simulink model "paper_Exponential_Predefined_102"  (R2019a)
settings: Solver=ode4  StartTime=0.0  StopTime=40  FixedStep=0.001  RelTol=1e-3
libraries: simulink x6
(part 1 of 3)
settings Model: Creator=maple  LastModifiedBy=maple

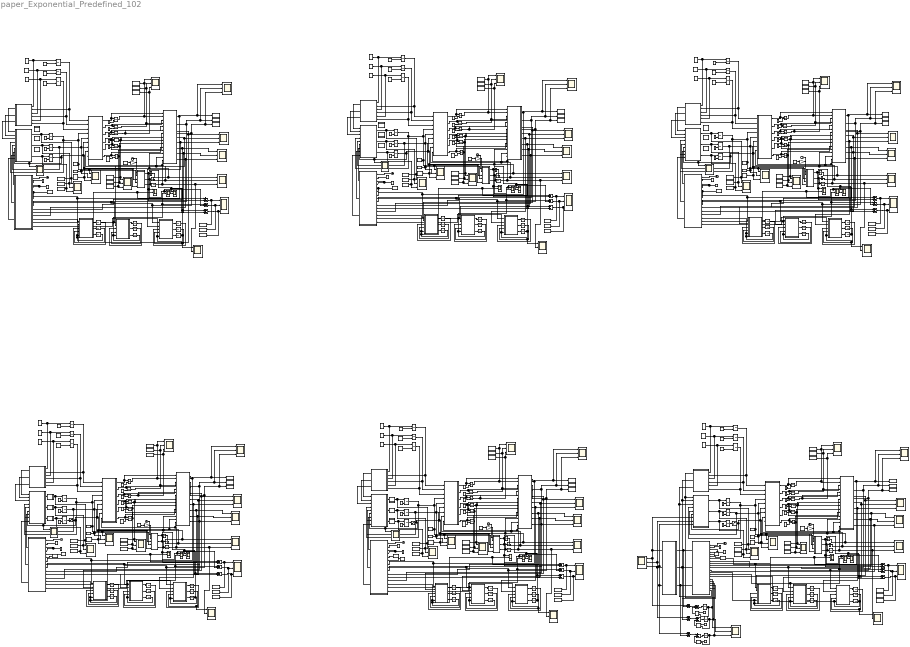
== system paper_Exponential_Predefined_102 ==
  note: p1z
  note: p2y
  note: p2z
  note: Predefined time in paper[11]
  note: p1x
  note: p2x
  note: p1y
  note: p1z
  note: p2z
  note: p1x
  note: Exponential predefined time
      | [This paper]
  note: p2y
  note: p2x
  note: p1y
  note: p1z
  note: p2z
  note: p1x
  note: p2y
  note: p2x
  note: p1y
  note: p2x
  note: tua1
  note: p1x
  note: p2z
  note: tua3
  note: p2y
  note: tua2
  note: p1y
  note: p1z
  note: p1y
  note: p2z
  note: p1z
  note: p1x
  note: Exponential
  note: p2x
  note: p2y
  note: p1z
  note: p2y
  note: p1x
  note: p2z
  note: p2x
  note: p1y
  note: Predefined time in paper[11]
  note: Exponential
  note: Exponential predefined time
      | [This paper]
  note: Without input saturation and disturbance
  note: With input saturation and disturbance
  " a^r1" : MATLAB Function  TreatAsAtomicUnit=on
  " a^r2" : MATLAB Function  TreatAsAtomicUnit=on
  " a^r3" : MATLAB Function  TreatAsAtomicUnit=on
  " a^r4" : MATLAB Function  TreatAsAtomicUnit=on
  " a^r5" : MATLAB Function  TreatAsAtomicUnit=on
  Add{1..15,39..47} (24 alike) : Sum  Inputs=+-
  Band-Limited White Noise{1..6} (6 alike) : simulink/Sources/Band-Limited White Noise  Cov=0.01  Ts=0.01  seed=[23341]
  Clock{1..6} (6 alike) : Clock
  Gain{1..6} (6 alike) : Gain  Gain=0.05
  MATLAB Function1 : MATLAB Function  TreatAsAtomicUnit=on
  MATLAB Function10 : MATLAB Function  TreatAsAtomicUnit=on
  MATLAB Function11 : MATLAB Function  TreatAsAtomicUnit=on
  MATLAB Function12 : MATLAB Function  TreatAsAtomicUnit=on
  MATLAB Function13 : MATLAB Function  TreatAsAtomicUnit=on
  MATLAB Function14 : MATLAB Function  TreatAsAtomicUnit=on
  MATLAB Function15 : MATLAB Function  TreatAsAtomicUnit=on
  MATLAB Function16 : MATLAB Function  TreatAsAtomicUnit=on
  MATLAB Function17 : MATLAB Function  TreatAsAtomicUnit=on
  MATLAB Function18 : MATLAB Function  TreatAsAtomicUnit=on
  MATLAB Function19 : MATLAB Function  TreatAsAtomicUnit=on
  MATLAB Function2 : MATLAB Function  TreatAsAtomicUnit=on
  MATLAB Function20 : MATLAB Function  TreatAsAtomicUnit=on
  MATLAB Function21 : MATLAB Function  TreatAsAtomicUnit=on
  MATLAB Function22 : MATLAB Function  TreatAsAtomicUnit=on
  MATLAB Function23 : MATLAB Function  TreatAsAtomicUnit=on
  MATLAB Function24 : MATLAB Function  TreatAsAtomicUnit=on
  MATLAB Function3 : MATLAB Function  TreatAsAtomicUnit=on
  MATLAB Function4 : MATLAB Function  TreatAsAtomicUnit=on
  MATLAB Function5 : MATLAB Function  TreatAsAtomicUnit=on
  MATLAB Function6 : MATLAB Function  TreatAsAtomicUnit=on
  MATLAB Function7 : MATLAB Function  TreatAsAtomicUnit=on
  MATLAB Function8 : MATLAB Function  TreatAsAtomicUnit=on
  MATLAB Function9 : MATLAB Function  TreatAsAtomicUnit=on
  Product13 : Product
  Product14 : Product
  Product15 : Product
  To Workspace1 : ToWorkspace  VariableName=deta  SampleTime=-1
  To Workspace10 : ToWorkspace  VariableName=x  SampleTime=-1
  To Workspace100 : ToWorkspace  VariableName=deta15  SampleTime=-1
  To Workspace101 : ToWorkspace  VariableName=y5  SampleTime=-1
  To Workspace102 : ToWorkspace  VariableName=p1x5  SampleTime=-1
  To Workspace103 : ToWorkspace  VariableName=p1y5  SampleTime=-1
  To Workspace104 : ToWorkspace  VariableName=xr5  SampleTime=-1
  To Workspace105 : ToWorkspace  VariableName=p1z5  SampleTime=-1
  To Workspace106 : ToWorkspace  VariableName=yr5  SampleTime=-1
  To Workspace107 : ToWorkspace  VariableName=z5  SampleTime=-1
  To Workspace108 : ToWorkspace  VariableName=zr5  SampleTime=-1
  To Workspace11 : ToWorkspace  VariableName=u  SampleTime=-1
  To Workspace12 : ToWorkspace  VariableName=u1  SampleTime=-1
  To Workspace13 : ToWorkspace  VariableName=u2  SampleTime=-1
  To Workspace14 : ToWorkspace  VariableName=psi  SampleTime=-1
  To Workspace15 : ToWorkspace  VariableName=gamma  SampleTime=-1
  To Workspace16 : ToWorkspace  VariableName=v  SampleTime=-1
  To Workspace17 : ToWorkspace  VariableName=deta1  SampleTime=-1
  To Workspace18 : ToWorkspace  VariableName=deta2  SampleTime=-1
  To Workspace19 : ToWorkspace  VariableName=deta3  SampleTime=-1
  To Workspace2 : ToWorkspace  VariableName=y  SampleTime=-1
  To Workspace20 : ToWorkspace  VariableName=x1  SampleTime=-1
  To Workspace21 : ToWorkspace  VariableName=u3  SampleTime=-1
  To Workspace22 : ToWorkspace  VariableName=u4  SampleTime=-1
  To Workspace23 : ToWorkspace  VariableName=u5  SampleTime=-1
  To Workspace24 : ToWorkspace  VariableName=psi1  SampleTime=-1
  To Workspace25 : ToWorkspace  VariableName=gamma1  SampleTime=-1
  To Workspace26 : ToWorkspace  VariableName=v1  SampleTime=-1
  To Workspace27 : ToWorkspace  VariableName=deta4  SampleTime=-1
  To Workspace28 : ToWorkspace  VariableName=deta5  SampleTime=-1
  To Workspace29 : ToWorkspace  VariableName=y1  SampleTime=-1
  To Workspace3 : ToWorkspace  VariableName=p1x  SampleTime=-1
  To Workspace30 : ToWorkspace  VariableName=p1x1  SampleTime=-1
  To Workspace31 : ToWorkspace  VariableName=p1y1  SampleTime=-1
  To Workspace32 : ToWorkspace  VariableName=xr1  SampleTime=-1
  To Workspace33 : ToWorkspace  VariableName=p1z1  SampleTime=-1
  To Workspace34 : ToWorkspace  VariableName=yr1  SampleTime=-1
  To Workspace35 : ToWorkspace  VariableName=z1  SampleTime=-1
  To Workspace36 : ToWorkspace  VariableName=zr1  SampleTime=-1
  To Workspace37 : ToWorkspace  VariableName=deta6  SampleTime=-1
  To Workspace38 : ToWorkspace  VariableName=x2  SampleTime=-1
  To Workspace39 : ToWorkspace  VariableName=u6  SampleTime=-1
  To Workspace4 : ToWorkspace  VariableName=p1y  SampleTime=-1
  To Workspace40 : ToWorkspace  VariableName=u7  SampleTime=-1
  To Workspace41 : ToWorkspace  VariableName=u8  SampleTime=-1
  To Workspace42 : ToWorkspace  VariableName=psi2  SampleTime=-1
  To Workspace43 : ToWorkspace  VariableName=gamma2  SampleTime=-1
  To Workspace44 : ToWorkspace  VariableName=v2  SampleTime=-1
  To Workspace45 : ToWorkspace  VariableName=deta7  SampleTime=-1
  To Workspace46 : ToWorkspace  VariableName=deta8  SampleTime=-1
  To Workspace47 : ToWorkspace  VariableName=y2  SampleTime=-1
  To Workspace48 : ToWorkspace  VariableName=p1x2  SampleTime=-1
  To Workspace49 : ToWorkspace  VariableName=p1y2  SampleTime=-1
  To Workspace5 : ToWorkspace  VariableName=xr  SampleTime=-1
  To Workspace50 : ToWorkspace  VariableName=xr2  SampleTime=-1
  To Workspace51 : ToWorkspace  VariableName=p1z2  SampleTime=-1
  To Workspace52 : ToWorkspace  VariableName=yr2  SampleTime=-1
  To Workspace53 : ToWorkspace  VariableName=z2  SampleTime=-1
  To Workspace54 : ToWorkspace  VariableName=zr2  SampleTime=-1
  To Workspace55 : ToWorkspace  VariableName=deta9  SampleTime=-1
  To Workspace56 : ToWorkspace  VariableName=x3  SampleTime=-1
  To Workspace57 : ToWorkspace  VariableName=u9  SampleTime=-1
  To Workspace58 : ToWorkspace  VariableName=u10  SampleTime=-1
  To Workspace59 : ToWorkspace  VariableName=u11  SampleTime=-1
  To Workspace6 : ToWorkspace  VariableName=p1z  SampleTime=-1
  To Workspace60 : ToWorkspace  VariableName=psi3  SampleTime=-1
  To Workspace61 : ToWorkspace  VariableName=gamma3  SampleTime=-1
  To Workspace62 : ToWorkspace  VariableName=v3  SampleTime=-1
  To Workspace63 : ToWorkspace  VariableName=deta10  SampleTime=-1
  To Workspace64 : ToWorkspace  VariableName=deta11  SampleTime=-1
  To Workspace65 : ToWorkspace  VariableName=y3  SampleTime=-1
  To Workspace66 : ToWorkspace  VariableName=p1x3  SampleTime=-1
  To Workspace67 : ToWorkspace  VariableName=p1y3  SampleTime=-1
  To Workspace68 : ToWorkspace  VariableName=xr3  SampleTime=-1
  To Workspace69 : ToWorkspace  VariableName=p1z3  SampleTime=-1
  To Workspace7 : ToWorkspace  VariableName=yr  SampleTime=-1
  To Workspace70 : ToWorkspace  VariableName=yr3  SampleTime=-1
  To Workspace71 : ToWorkspace  VariableName=z3  SampleTime=-1
  To Workspace72 : ToWorkspace  VariableName=zr3  SampleTime=-1
  To Workspace73 : ToWorkspace  VariableName=deta12  SampleTime=-1
  To Workspace74 : ToWorkspace  VariableName=x4  SampleTime=-1
  To Workspace75 : ToWorkspace  VariableName=u12  SampleTime=-1
  To Workspace76 : ToWorkspace  VariableName=u13  SampleTime=-1
  To Workspace77 : ToWorkspace  VariableName=u14  SampleTime=-1
  To Workspace78 : ToWorkspace  VariableName=psi4  SampleTime=-1
  To Workspace79 : ToWorkspace  VariableName=gamma4  SampleTime=-1
  To Workspace8 : ToWorkspace  VariableName=z  SampleTime=-1
  To Workspace80 : ToWorkspace  VariableName=v4  SampleTime=-1
  To Workspace81 : ToWorkspace  VariableName=deta13  SampleTime=-1
  To Workspace82 : ToWorkspace  VariableName=deta14  SampleTime=-1
  To Workspace83 : ToWorkspace  VariableName=y4  SampleTime=-1
  To Workspace84 : ToWorkspace  VariableName=p1x4  SampleTime=-1
  To Workspace85 : ToWorkspace  VariableName=p1y4  SampleTime=-1
  To Workspace86 : ToWorkspace  VariableName=xr4  SampleTime=-1
  To Workspace87 : ToWorkspace  VariableName=p1z4  SampleTime=-1
  To Workspace88 : ToWorkspace  VariableName=yr4  SampleTime=-1
  To Workspace89 : ToWorkspace  VariableName=z4  SampleTime=-1
  To Workspace9 : ToWorkspace  VariableName=zr  SampleTime=-1
  To Workspace90 : ToWorkspace  VariableName=zr4  SampleTime=-1
  To Workspace91 : ToWorkspace  VariableName=x5  SampleTime=-1
  To Workspace92 : ToWorkspace  VariableName=u15  SampleTime=-1
  To Workspace93 : ToWorkspace  VariableName=u16  SampleTime=-1
  To Workspace94 : ToWorkspace  VariableName=u17  SampleTime=-1
  To Workspace95 : ToWorkspace  VariableName=psi5  SampleTime=-1
  To Workspace96 : ToWorkspace  VariableName=gamma5  SampleTime=-1
  To Workspace97 : ToWorkspace  VariableName=v5  SampleTime=-1
  To Workspace98 : ToWorkspace  VariableName=deta16  SampleTime=-1
  To Workspace99 : ToWorkspace  VariableName=deta17  SampleTime=-1
  U : MATLAB Function  TreatAsAtomicUnit=on
  X{1..5} (5 alike) : Scope  NumInputPorts=3
  X_dot1 : MATLAB Function  TreatAsAtomicUnit=on
  X_dot2 : MATLAB Function  TreatAsAtomicUnit=on
  X_dot3 : MATLAB Function  TreatAsAtomicUnit=on
  X_dot4 : MATLAB Function  TreatAsAtomicUnit=on
  X_dot5 : MATLAB Function  TreatAsAtomicUnit=on
  X_dot6 : MATLAB Function  TreatAsAtomicUnit=on
  ar{1..6} (6 alike) : Constant  Value=0
  bta{1..6} (6 alike) : Constant  Value=6
  control input 1 : MATLAB Function  TreatAsAtomicUnit=on
  control input 2 : MATLAB Function  TreatAsAtomicUnit=on
  control input 3 : MATLAB Function  TreatAsAtomicUnit=on
  control input 4 : MATLAB Function  TreatAsAtomicUnit=on
  control input 5 : MATLAB Function  TreatAsAtomicUnit=on
  d2x {1..6} (6 alike) : Integrator
  d2y {1..6} (6 alike) : Integrator
  d2z {1..6} (6 alike) : Integrator
  error_FTDO1 : Scope  NumInputPorts=3
  error_FTDO2 : Scope  NumInputPorts=3
  f,df1 : MATLAB Function  TreatAsAtomicUnit=on
  f,df2 : MATLAB Function  TreatAsAtomicUnit=on
  f,df3 : MATLAB Function  TreatAsAtomicUnit=on
  f,df4 : MATLAB Function  TreatAsAtomicUnit=on
  f,df5 : MATLAB Function  TreatAsAtomicUnit=on
  gamma{1,3,5,7,9,11} (6 alike) : Constant  Value=0
  gamma{2,4,6,8,10,12} (6 alike) : Integrator  InitialConditionSource=external
  gamma_r{1,3,5,7,9,11} (6 alike) : Integrator  InitialConditionSource=external
  gamma_r{2,4,6,8,10,12} (6 alike) : Constant  Value=0.2
  k{1..2,4..5,8,18} (6 alike) : Constant
  k19 : Constant  Value=3
  k20 : Constant  Value=3
  k21 : Constant  Value=3
  k3 : Constant  Value=0.3
  k7 : Constant  Value=0.3
  k9 : Constant  Value=0.3
  omiga__gamma_r{1..6} (6 alike) : Constant  Value=0
  omiga_psi_r{1..6} (6 alike) : Constant  Value=0.3
  p{1..28,35..36} (30 alike) : Scope  NumInputPorts=3
  predefined : MATLAB Function  TreatAsAtomicUnit=on
  psi{1,3,5,7,9,11} (6 alike) : Constant  Value=0
  psi{2,4,6,8,10,12} (6 alike) : Integrator  InitialConditionSource=external
  psi_r{1,3,5,7,9} (5 alike) : Constant  Value=3.14/4
  psi_r{2,4,6,8,10,12} (6 alike) : Integrator  InitialConditionSource=external
  psi_r11 : Constant  Value=0.3
  qnta : MATLAB Function  TreatAsAtomicUnit=on
  real_disturbance : Scope  NumInputPorts=3
  ref_UAV : MATLAB Function  TreatAsAtomicUnit=on
  reference_position : Scope  NumInputPorts=3
  sat_v1 : Saturate  UpperLimit=30  LowerLimit=10
  sat_v2 : Saturate  UpperLimit=30  LowerLimit=10
  sat_v6 : Saturate  UpperLimit=40  LowerLimit=10
  show Xr{1..5} (5 alike) : Scope  NumInputPorts=3
  show_p1 : Scope  NumInputPorts=3
  show_p2 : Scope  NumInputPorts=3
  show_qnta : Scope  NumInputPorts=3
  show_s : Scope  NumInputPorts=3
  show_tua : Scope  NumInputPorts=3
  show_u{,1..10} (11 alike) : Scope  NumInputPorts=3
  show_v psi gamma{1..24} (24 alike) : Scope  NumInputPorts=3
  sys : MATLAB Function  TreatAsAtomicUnit=on
  t{1..6} (6 alike) : Clock
  t_f1 : Constant  Value=5
  t_f2 : Constant  Value=5
  t_f3 : Constant  Value=20
  t_f4 : Constant  Value=5
  t_f5 : Constant  Value=20
  t_f6 : Constant  Value=20
  tua13 : Integrator
  tua14 : Integrator
  tua15 : Integrator
  u_1a1 : MATLAB Function  TreatAsAtomicUnit=on
  u_1a2 : MATLAB Function  TreatAsAtomicUnit=on
  u_1a3 : MATLAB Function  TreatAsAtomicUnit=on
  u_1a4 : MATLAB Function  TreatAsAtomicUnit=on
  u_1a5 : MATLAB Function  TreatAsAtomicUnit=on
  u_2a1 : MATLAB Function  TreatAsAtomicUnit=on
  u_2a2 : MATLAB Function  TreatAsAtomicUnit=on
  u_2a3 : MATLAB Function  TreatAsAtomicUnit=on
  u_2a4 : MATLAB Function  TreatAsAtomicUnit=on
  u_2a6 : MATLAB Function  TreatAsAtomicUnit=on
  u_3a1 : MATLAB Function  TreatAsAtomicUnit=on
  u_3a2 : MATLAB Function  TreatAsAtomicUnit=on
  u_3a3 : MATLAB Function  TreatAsAtomicUnit=on
  u_3a4 : MATLAB Function  TreatAsAtomicUnit=on
  u_3a5 : MATLAB Function  TreatAsAtomicUnit=on
  uav_position : Scope  NumInputPorts=3
  v{1,3,5,7,9,11} (6 alike) : Constant  Value=10
  v{2,4,6,8,10,12} (6 alike) : Integrator  InitialConditionSource=external
  vr{1,3,5,7,9,11} (6 alike) : Constant  Value=20
  vr{2,4,6,8,10,12} (6 alike) : Integrator  InitialConditionSource=external
  x{1,3,5,7,9,11} (6 alike) : Constant  Value=0
  x{2,4,6,8,10,12} (6 alike) : Integrator  InitialConditionSource=external
  xr{1,3,5,7,9,11} (6 alike) : Constant  Value=70
  xr{2,4,6,8,10,12} (6 alike) : Integrator  InitialConditionSource=external
  y{1,3,5,7,9,11} (6 alike) : Constant  Value=0
  y{2,4,6,8,10,12} (6 alike) : Integrator  InitialConditionSource=external
  yr{1,3,5,7,9,11} (6 alike) : Constant  Value=90
  yr{2,4,6,8,10,12} (6 alike) : Integrator  InitialConditionSource=external
  yuding_zhishu1 : MATLAB Function  TreatAsAtomicUnit=on
  yuding_zhishu2 : MATLAB Function  TreatAsAtomicUnit=on
  yuding_zhishu3 : MATLAB Function  TreatAsAtomicUnit=on
  yuding_zhishu4 : MATLAB Function  TreatAsAtomicUnit=on
  yuding_zhishu5 : MATLAB Function  TreatAsAtomicUnit=on
  z0x{1..6} (6 alike) : Integrator  InitialCondition=70
  z0y{1..6} (6 alike) : Integrator  InitialCondition=90
  z0z{1..6} (6 alike) : Integrator  InitialCondition=-100
  z{1,3,5,7,9,11} (6 alike) : Constant  Value=0
  z{2,4,6,8,10,12} (6 alike) : Integrator  InitialConditionSource=external
  z1x{1..6} (6 alike) : Integrator
  z1y{1..6} (6 alike) : Integrator
  z1z{1..6} (6 alike) : Integrator
  z2x{1..6} (6 alike) : Integrator
  z2y{1..6} (6 alike) : Integrator
  z2z{1..6} (6 alike) : Integrator
  zr{1,3,5,7,9,11} (6 alike) : Constant  Value=-100
  zr{2,4,6,8,10,12} (6 alike) : Integrator  InitialConditionSource=external
  wires:
  yr2/1 -> To Workspace7/1, show Xr1/2, f,df1/10(yr)
  zr2/1 -> To Workspace9/1, show Xr1/3, f,df1/12(zr)
  MATLAB Function1/1(dz0y) -> z0y1/1
  d2y 1/1 -> p6/2, f,df1/14(wy), X_dot1/8(wy)
  MATLAB Function4/1(dz0x) -> z0x1/1
  t1/1 -> yuding_zhishu1/1(t)
  " a^r1"/1(a_xr) -> control input 1/1(a_xr)
  omiga__gamma_r1/1 -> " a^r1"/5(omiga_gamma_r), gamma_r1/1
  f,df1/2(p1y) -> MATLAB Function1/1(p1y), yuding_zhishu1/8(p1y), To Workspace4/1, p4/2
  z0y1/1 -> MATLAB Function1/3(z0y)
  f,df1/5(p2y) -> MATLAB Function1/2(p2y), p5/2
  X_dot1/4(xr_dot) -> f,df1/7(dxr), xr2/1
  Band-Limited White Noise1/1 -> Gain1/1
  x2/1 -> To Workspace10/1, X1/1, f,df1/2(x)
  MATLAB Function3/2(dz1z) -> z1z1/1
  " a^r1"/3(a_zr) -> control input 1/3(a_zr)
  z0x1/1 -> MATLAB Function4/3(z0x)
  d2x 1/1 -> f,df1/13(wx), X_dot1/7(wx), p6/1
  xr1/1 -> xr2/2
  gamma2/1 -> MATLAB Function2/4(gamma), show_v psi gamma4/2, To Workspace15/1, X_dot1/5(gamma), control input 1/5(gamma)
  z2/1 -> To Workspace8/1, X1/3, f,df1/6(z)
  psi2/1 -> To Workspace14/1, show_v psi gamma4/1, MATLAB Function2/5(psi), X_dot1/4(psi), control input 1/4(psi)
  MATLAB Function4/2(dz1x) -> z1x1/1
  MATLAB Function4/3(dz2x) -> z2x1/1
  MATLAB Function2/1(dx) -> Add3/2, show_v psi gamma1/1, d2x 1/1
  xr2/1 -> To Workspace5/1, show Xr1/1, f,df1/8(xr)
  z1x1/1 -> MATLAB Function4/4(z1x)
  z1y1/1 -> MATLAB Function1/4(z1y)
  bta1/1 -> yuding_zhishu1/4(bta2), yuding_zhishu1/3(bta1)
  k1/1 -> yuding_zhishu1/6(k2), yuding_zhishu1/5(k1)
  z1z1/1 -> MATLAB Function3/4(z1z), p2/1
  X_dot1/1(s1) -> f,df1/1(dx), x2/1
  f,df1/1(p1x) -> MATLAB Function4/1(p1x), yuding_zhishu1/7(p1x), To Workspace3/1, p4/1
  Clock1/1 -> MATLAB Function2/1(t)
  x1/1 -> x2/2
  psi_r1/1 -> psi_r2/2
  gamma_r1/1 -> " a^r1"/6(gamma_r), X_dot1/3(gamma_r)
  z2y1/1 -> MATLAB Function1/5(z2y), Add4/1, show_v psi gamma2/2, yuding_zhishu1/14(z2y)
  f,df1/8(s2) -> yuding_zhishu1/11(p2y), p3/2
  d2z 1/1 -> f,df1/15(wz), X_dot1/9(wz), p2/2, p6/3
  f,df1/3(p1z) -> MATLAB Function3/1(p1z), yuding_zhishu1/9(p1z), To Workspace6/1, p4/3
  Add5/1 -> To Workspace1/1, p1/3
  t_f1/1 -> yuding_zhishu1/2(t_f)
  f,df1/6(p2z) -> MATLAB Function3/2(p2z), p5/3
  X_dot1/6(zr_dot) -> f,df1/11(dzr), zr2/1
  gamma_r2/1 -> gamma_r1/2
  MATLAB Function1/2(dz1y) -> z1y1/1
  z2z1/1 -> Add5/1, show_v psi gamma3/2, MATLAB Function3/5(z2z), yuding_zhishu1/15(z2z)
  X_dot1/5(yr_dot) -> yr2/1, f,df1/9(dyr)
  z2x1/1 -> Add3/1, show_v psi gamma1/2, MATLAB Function4/5(z2x), yuding_zhishu1/13(z2x)
  vr2/1 -> X_dot1/1(vr), " a^r1"/2(vr)
  ar1/1 -> " a^r1"/1(ar), vr2/1
  MATLAB Function2/2(dy) -> d2y 1/1, Add4/2, show_v psi gamma2/1
  psi_r2/1 -> X_dot1/2(psi_r), " a^r1"/4(psi_r)
  omiga_psi_r1/1 -> " a^r1"/3(omiga_psi_r), psi_r2/1
  y2/1 -> To Workspace2/1, X1/2, f,df1/4(y)
  f,df1/4(p2x) -> MATLAB Function4/2(p2x), p5/1
  MATLAB Function3/1(dz0z) -> z0z1/1
  vr1/1 -> vr2/2
  y1/1 -> y2/2
  " a^r1"/2(a_yr) -> control input 1/2(a_yr)
  f,df1/9(s3) -> yuding_zhishu1/12(p2z), p3/3
  psi1/1 -> psi2/2
  z0z1/1 -> MATLAB Function3/3(z0z)
  Add3/1 -> To Workspace17/1, p1/1
  MATLAB Function3/3(dz2z) -> z2z1/1
  v2/1 -> MATLAB Function2/3(v), To Workspace16/1, show_v psi gamma4/3, X_dot1/6(v), show_u2/1, control input 1/6(v)
  z1/1 -> z2/2
  MATLAB Function1/3(dz2y) -> z2y1/1
  yr1/1 -> yr2/2
  v1/1 -> v2/2
  Gain1/1 -> MATLAB Function2/2(delta)
  X_dot1/2(s2) -> y2/1, f,df1/3(dy)
  gamma1/1 -> gamma2/2
  zr1/1 -> zr2/2
  Add4/1 -> To Workspace18/1, p1/2
  X_dot1/3(s3) -> f,df1/5(dz), z2/1
  f,df1/7(s1) -> yuding_zhishu1/10(p2x), p3/1
  MATLAB Function2/3(dz) -> Add5/2, show_v psi gamma3/1, d2z 1/1
  yuding_zhishu1/1(nta_1) -> control input 1/7(nta_1)
  yuding_zhishu1/2(nta_2) -> control input 1/8(nta_2)
  yuding_zhishu1/3(nta_3) -> control input 1/9(nta_3)
  control input 1/3(u3_a) -> v2/1, To Workspace13/1, show_u1/3
  control input 1/2(u2_omiga_gamma) -> To Workspace12/1, show_u1/2, gamma2/1
  control input 1/1(u1_omiga_psi) -> psi2/1, To Workspace11/1, show_u1/1
  gamma_r3/1 -> " a^r2"/6(gamma_r), X_dot2/3(gamma_r)
  z2y2/1 -> Add2/1, show_v psi gamma6/2, yuding_zhishu2/14(z2y), MATLAB Function5/5(z2y)
  psi_r3/1 -> psi_r4/2
  z0x2/1 -> MATLAB Function8/3(z0x)
  MATLAB Function7/3(dz2z) -> z2z2/1
  y4/1 -> To Workspace29/1, X2/2, f,df2/4(y)
  gamma3/1 -> gamma4/2
  control input 2/1(u1_omiga_psi) -> psi4/1, To Workspace21/1, show_u3/1
  v4/1 -> MATLAB Function6/3(v), To Workspace26/1, show_v psi gamma8/3, X_dot2/6(v), show_u4/1, control input 2/6(v)
  f,df2/6(p2z) -> MATLAB Function7/2(p2z), p11/3
  yuding_zhishu2/3(nta_3) -> control input 2/9(nta_3)
  control input 2/2(u2_omiga_gamma) -> To Workspace22/1, show_u3/2, gamma4/1
  f,df2/7(s1) -> yuding_zhishu2/10(p2x), p9/1
  gamma_r4/1 -> gamma_r3/2
  control input 2/3(u3_a) -> v4/1, To Workspace23/1, show_u3/3
  yuding_zhishu2/2(nta_2) -> control input 2/8(nta_2)
  f,df2/8(s2) -> yuding_zhishu2/11(p2y), p9/2
  z3/1 -> z4/2
  Add2/1 -> To Workspace28/1, p7/2
  yuding_zhishu2/1(nta_1) -> control input 2/7(nta_1)
  MATLAB Function6/3(dz) -> Add6/2, show_v psi gamma7/1, d2z 2/1
  yr3/1 -> yr4/2
  zr3/1 -> zr4/2
  z1y2/1 -> MATLAB Function5/4(z1y)
  X_dot2/2(s2) -> y4/1, f,df2/3(dy)
  X_dot2/3(s3) -> f,df2/5(dz), z4/1
  " a^r2"/2(a_yr) -> control input 2/2(a_yr)
  Band-Limited White Noise2/1 -> Gain2/1
  Add6/1 -> To Workspace19/1, p7/3
  y3/1 -> y4/2
  Add1/1 -> To Workspace27/1, p7/1
  Gain2/1 -> MATLAB Function6/2(delta)
  MATLAB Function8/2(dz1x) -> z1x2/1
  f,df2/2(p1y) -> MATLAB Function5/1(p1y), yuding_zhishu2/8(p1y), To Workspace31/1, p10/2
  MATLAB Function5/3(dz2y) -> z2y2/1
  psi3/1 -> psi4/2
  z0z2/1 -> MATLAB Function7/3(z0z)
  z2z2/1 -> Add6/1, show_v psi gamma7/2, yuding_zhishu2/15(z2z), MATLAB Function7/5(z2z)
  f,df2/9(s3) -> yuding_zhishu2/12(p2z), p9/3
  vr3/1 -> vr4/2
  psi_r4/1 -> X_dot2/2(psi_r), " a^r2"/4(psi_r)
  z1z2/1 -> p8/1, MATLAB Function7/4(z1z)
  MATLAB Function6/1(dx) -> Add1/2, show_v psi gamma5/1, d2x 2/1
  MATLAB Function8/3(dz2x) -> z2x2/1
  xr3/1 -> xr4/2
  z0y2/1 -> MATLAB Function5/3(z0y)
  t2/1 -> yuding_zhishu2/1(t)
  MATLAB Function7/2(dz1z) -> z1z2/1
  d2x 2/1 -> f,df2/13(wx), X_dot2/7(wx), p12/1
  MATLAB Function8/1(dz0x) -> z0x2/1
  omiga__gamma_r2/1 -> " a^r2"/5(omiga_gamma_r), gamma_r3/1
  " a^r2"/1(a_xr) -> control input 2/1(a_xr)
  MATLAB Function5/1(dz0y) -> z0y2/1
  yr4/1 -> To Workspace34/1, show Xr2/2, f,df2/10(yr)
  zr4/1 -> To Workspace36/1, show Xr2/3, f,df2/12(zr)
  v3/1 -> v4/2
  bta2/1 -> yuding_zhishu2/4(bta2), yuding_zhishu2/3(bta1)
  d2y 2/1 -> p12/2, f,df2/14(wy), X_dot2/8(wy)
  psi4/1 -> To Workspace24/1, show_v psi gamma8/1, MATLAB Function6/5(psi), X_dot2/4(psi), control input 2/4(psi)
  z1x2/1 -> MATLAB Function8/4(z1x)
  MATLAB Function7/1(dz0z) -> z0z2/1
  z4/1 -> To Workspace35/1, X2/3, f,df2/6(z)
  gamma4/1 -> MATLAB Function6/4(gamma), show_v psi gamma8/2, To Workspace25/1, X_dot2/5(gamma), control input 2/5(gamma)
  " a^r2"/3(a_zr) -> control input 2/3(a_zr)
  X_dot2/6(zr_dot) -> f,df2/11(dzr), zr4/1
  omiga_psi_r2/1 -> " a^r2"/3(omiga_psi_r), psi_r4/1
  f,df2/1(p1x) -> MATLAB Function8/1(p1x), yuding_zhishu2/7(p1x), To Workspace30/1, p10/1
  f,df2/4(p2x) -> MATLAB Function8/2(p2x), p11/1
  X_dot2/1(s1) -> f,df2/1(dx), x4/1
  x3/1 -> x4/2
  z2x2/1 -> Add1/1, show_v psi gamma5/2, yuding_zhishu2/13(z2x), MATLAB Function8/5(z2x)
  X_dot2/4(xr_dot) -> f,df2/7(dxr), xr4/1
  vr4/1 -> X_dot2/1(vr), " a^r2"/2(vr)
  x4/1 -> To Workspace20/1, X2/1, f,df2/2(x)
  xr4/1 -> To Workspace32/1, show Xr2/1, f,df2/8(xr)
  f,df2/3(p1z) -> MATLAB Function7/1(p1z), yuding_zhishu2/9(p1z), To Workspace33/1, p10/3
  X_dot2/5(yr_dot) -> yr4/1, f,df2/9(dyr)
  k2/1 -> yuding_zhishu2/6(k2), yuding_zhishu2/5(k1)
  f,df2/5(p2y) -> MATLAB Function5/2(p2y), p11/2
  Clock2/1 -> MATLAB Function6/1(t)
  t_f2/1 -> yuding_zhishu2/2(t_f)
  ar2/1 -> " a^r2"/1(ar), vr4/1
  MATLAB Function6/2(dy) -> d2y 2/1, Add2/2, show_v psi gamma6/1
  d2z 2/1 -> f,df2/15(wz), X_dot2/9(wz), p8/2, p12/3
  MATLAB Function5/2(dz1y) -> z1y2/1
  gamma_r5/1 -> " a^r3"/6(gamma_r), X_dot3/3(gamma_r)
  z2y3/1 -> Add8/1, show_v psi gamma10/2, yuding_zhishu3/14(z2y), MATLAB Function9/5(z2y)
  psi_r5/1 -> psi_r6/2
  z0x3/1 -> MATLAB Function12/3(z0x)
  MATLAB Function11/3(dz2z) -> z2z3/1
  y6/1 -> To Workspace47/1, X3/2, f,df3/4(y)
  gamma5/1 -> gamma6/2
  control input 3/1(u1_omiga_psi) -> u_1a3/1(u)
  v6/1 -> sat_v1/1
  f,df3/6(p2z) -> MATLAB Function11/2(p2z), p17/3
  yuding_zhishu3/3(nta_3) -> control input 3/9(nta_3)
  control input 3/2(u2_omiga_gamma) -> u_2a3/1(u)
  f,df3/7(s1) -> yuding_zhishu3/10(p2x), p15/1
  gamma_r6/1 -> gamma_r5/2
  control input 3/3(u3_a) -> u_3a3/1(u)
  yuding_zhishu3/2(nta_2) -> control input 3/8(nta_2)
  f,df3/8(s2) -> yuding_zhishu3/11(p2y), p15/2
  z5/1 -> z6/2
  Add8/1 -> To Workspace46/1, p13/2
  yuding_zhishu3/1(nta_1) -> control input 3/7(nta_1)
  MATLAB Function10/3(dz) -> Add9/2, show_v psi gamma11/1, d2z 3/1
  yr5/1 -> yr6/2
  zr5/1 -> zr6/2
  z1y3/1 -> MATLAB Function9/4(z1y)
  X_dot3/2(s2) -> y6/1, f,df3/3(dy)
  X_dot3/3(s3) -> f,df3/5(dz), z6/1
  " a^r3"/2(a_yr) -> control input 3/2(a_yr)
  Band-Limited White Noise3/1 -> Gain3/1
  Add9/1 -> To Workspace37/1, p13/3
  y5/1 -> y6/2
  Add7/1 -> To Workspace45/1, p13/1
  Gain3/1 -> MATLAB Function10/2(delta)
  MATLAB Function12/2(dz1x) -> z1x3/1
  f,df3/2(p1y) -> MATLAB Function9/1(p1y), yuding_zhishu3/8(p1y), To Workspace49/1, p16/2
  MATLAB Function9/3(dz2y) -> z2y3/1
  psi5/1 -> psi6/2
  z0z3/1 -> MATLAB Function11/3(z0z)
  z2z3/1 -> Add9/1, show_v psi gamma11/2, yuding_zhishu3/15(z2z), MATLAB Function11/5(z2z)
  f,df3/9(s3) -> yuding_zhishu3/12(p2z), p15/3
  vr5/1 -> vr6/2
  psi_r6/1 -> X_dot3/2(psi_r), " a^r3"/4(psi_r)
  z1z3/1 -> p14/1, MATLAB Function11/4(z1z)
  MATLAB Function10/1(dx) -> Add7/2, show_v psi gamma9/1, d2x 3/1
  MATLAB Function12/3(dz2x) -> z2x3/1
  xr5/1 -> xr6/2
  z0y3/1 -> MATLAB Function9/3(z0y)
  t3/1 -> yuding_zhishu3/1(t)
  MATLAB Function11/2(dz1z) -> z1z3/1
  d2x 3/1 -> f,df3/13(wx), X_dot3/7(wx), p18/1
  MATLAB Function12/1(dz0x) -> z0x3/1
  omiga__gamma_r3/1 -> " a^r3"/5(omiga_gamma_r), gamma_r5/1
  " a^r3"/1(a_xr) -> control input 3/1(a_xr)
  MATLAB Function9/1(dz0y) -> z0y3/1
  yr6/1 -> To Workspace52/1, show Xr3/2, f,df3/10(yr)
  zr6/1 -> To Workspace54/1, show Xr3/3, f,df3/12(zr)
  v5/1 -> v6/2
  bta3/1 -> yuding_zhishu3/4(bta2), yuding_zhishu3/3(bta1)
  d2y 3/1 -> p18/2, f,df3/14(wy), X_dot3/8(wy)
  psi6/1 -> To Workspace42/1, show_v psi gamma12/1, MATLAB Function10/5(psi), X_dot3/4(psi), control input 3/4(psi)
  z1x3/1 -> MATLAB Function12/4(z1x)
  MATLAB Function11/1(dz0z) -> z0z3/1
  z6/1 -> To Workspace53/1, X3/3, f,df3/6(z)
  gamma6/1 -> MATLAB Function10/4(gamma), show_v psi gamma12/2, To Workspace43/1, X_dot3/5(gamma), control input 3/5(gamma)
  " a^r3"/3(a_zr) -> control input 3/3(a_zr)
  X_dot3/6(zr_dot) -> f,df3/11(dzr), zr6/1
  omiga_psi_r3/1 -> " a^r3"/3(omiga_psi_r), psi_r6/1
  f,df3/1(p1x) -> MATLAB Function12/1(p1x), yuding_zhishu3/7(p1x), To Workspace48/1, p16/1
  f,df3/4(p2x) -> MATLAB Function12/2(p2x), p17/1
  X_dot3/1(s1) -> f,df3/1(dx), x6/1
  x5/1 -> x6/2
  z2x3/1 -> Add7/1, show_v psi gamma9/2, yuding_zhishu3/13(z2x), MATLAB Function12/5(z2x)
  X_dot3/4(xr_dot) -> f,df3/7(dxr), xr6/1
  vr6/1 -> X_dot3/1(vr), " a^r3"/2(vr)
  x6/1 -> To Workspace38/1, X3/1, f,df3/2(x)
  xr6/1 -> To Workspace50/1, show Xr3/1, f,df3/8(xr)
  f,df3/3(p1z) -> MATLAB Function11/1(p1z), yuding_zhishu3/9(p1z), To Workspace51/1, p16/3
  X_dot3/5(yr_dot) -> yr6/1, f,df3/9(dyr)
  k3/1 -> yuding_zhishu3/5(k1)
  f,df3/5(p2y) -> MATLAB Function9/2(p2y), p17/2
  Clock3/1 -> MATLAB Function10/1(t)
  t_f3/1 -> yuding_zhishu3/2(t_f)
  ar3/1 -> " a^r3"/1(ar), vr6/1
  MATLAB Function10/2(dy) -> d2y 3/1, Add8/2, show_v psi gamma10/1
  d2z 3/1 -> f,df3/15(wz), X_dot3/9(wz), p14/2, p18/3
  MATLAB Function9/2(dz1y) -> z1y3/1
  sat_v1/1 -> MATLAB Function10/3(v), To Workspace44/1, show_v psi gamma12/3, X_dot3/6(v), show_u6/1, control input 3/6(v)
  u_3a3/1(u_3a) -> v6/1, To Workspace41/1, show_u5/3
  u_2a3/1(u_2a) -> To Workspace40/1, show_u5/2, gamma6/1
  u_1a3/1(u_1a) -> psi6/1, To Workspace39/1, show_u5/1
  Band-Limited White Noise6/1 -> Gain6/1
  tua15/1 -> Product15/2, show_tua/3, predefined/18(tua3)
  k19/1 -> Product14/1
  Add44/1 -> Add45/1
  psi11/1 -> psi12/2
  Clock6/1 -> MATLAB Function22/1(t)
  vr12/1 -> X_dot6/1(vr), ref_UAV/2(vr)
  z12/1 -> To Workspace107/1, uav_position/3, sys/6(z)
  t6/1 -> predefined/1(t)
  X_dot6/4(xr_dot) -> sys/7(dxr), xr12/1
  Add47/1 -> tua14/1
  X_dot6/6(zr_dot) -> sys/11(dzr), zr12/1
  MATLAB Function21/1(dz0y) -> z0y6/1
  Product15/1 -> Add40/2
  z0z6/1 -> MATLAB Function23/3(z0z)
  zr12/1 -> To Workspace108/1, reference_position/3, sys/12(zr)
  x11/1 -> x12/2
  z0y6/1 -> MATLAB Function21/3(z0y)
  Add43/1 -> To Workspace100/1, error_FTDO1/3
  sys/7(s1) -> show_s/1, predefined/10(p2x)
  t_f6/1 -> predefined/2(t_f)
  y12/1 -> To Workspace101/1, uav_position/2, sys/4(y)
  Add41/1 -> To Workspace98/1, error_FTDO1/1
  sys/4(p2x) -> MATLAB Function24/2(p2x), show_p2/1
  MATLAB Function22/3(dz) -> Add43/2, show_v psi gamma23/1, d2z 5/1
  Add42/1 -> To Workspace99/1, error_FTDO1/2
  Add39/1 -> Add40/1
  Product14/1 -> Add47/2
  MATLAB Function21/3(dz2y) -> z2y6/1
  z1z6/1 -> error_FTDO2/1, MATLAB Function23/4(z1z)
  v12/1 -> sat_v6/1
  d2x 6/1 -> sys/13(wx), X_dot6/7(wx), real_disturbance/1
  ref_UAV/1(a_xr) -> U/1(a_xr), predefined/19(a_xr)
  sys/3(p1z) -> MATLAB Function23/1(p1z), predefined/9(p1z), To Workspace105/1, show_p1/3
  omiga__gamma_r6/1 -> ref_UAV/5(omiga_gamma_r), gamma_r11/1
  v11/1 -> v12/2
  MATLAB Function21/2(dz1y) -> z1y6/1
  y11/1 -> y12/2
  qnta/3(qnta3) -> Add39/1, U/9(qnta_3), show_qnta/3
  k20/1 -> Product13/1
  z1x6/1 -> MATLAB Function24/4(z1x)
  d2z 5/1 -> sys/15(wz), X_dot6/9(wz), error_FTDO2/2, real_disturbance/3
  z11/1 -> z12/2
  Add40/1 -> tua15/1
  MATLAB Function23/3(dz2z) -> z2z6/1
  sys/6(p2z) -> MATLAB Function23/2(p2z), show_p2/3
  Gain6/1 -> MATLAB Function22/2(delta)
  xr11/1 -> xr12/2
  MATLAB Function23/2(dz1z) -> z1z6/1
  gamma11/1 -> gamma12/2
  yr12/1 -> To Workspace106/1, reference_position/2, sys/10(yr)
  X_dot6/2(dy) -> y12/1, sys/3(dy)
  ref_UAV/3(a_zr) -> U/3(a_zr), predefined/21(a_zr)
  vr11/1 -> vr12/2
  predefined/1(nta_1) -> qnta/1(nta1), Add44/2
  d2y 6/1 -> real_disturbance/2, sys/14(wy), X_dot6/8(wy)
  yr11/1 -> yr12/2
  MATLAB Function24/3(dz2x) -> z2x6/1
  qnta/1(qnta1) -> show_qnta/1, Add44/1, U/7(qnta_1)
  psi_r12/1 -> X_dot6/2(psi_r), ref_UAV/4(psi_r)
  U/1(u1_omiga_psi) -> psi12/1, To Workspace92/1, show_u/1
  MATLAB Function24/1(dz0x) -> z0x6/1
  xr12/1 -> To Workspace104/1, reference_position/1, sys/8(xr)
  sat_v6/1 -> MATLAB Function22/3(v), To Workspace97/1, show_v psi gamma24/3, X_dot6/6(v), U/6(v)
  MATLAB Function24/2(dz1x) -> z1x6/1
  bta6/1 -> predefined/4(bta2), predefined/3(bta1)
  sys/5(p2y) -> MATLAB Function21/2(p2y), show_p2/2
  Product13/1 -> Add45/2
  z2x6/1 -> Add41/1, show_v psi gamma21/2, predefined/13(z2x), MATLAB Function24/5(z2x)
  MATLAB Function23/1(dz0z) -> z0z6/1
  ar6/1 -> ref_UAV/1(ar), vr12/1
  tua13/1 -> show_tua/1, predefined/16(tua1), Product13/2
  X_dot6/5(yr_dot) -> yr12/1, sys/9(dyr)
  sys/1(p1x) -> MATLAB Function24/1(p1x), predefined/7(p1x), To Workspace102/1, show_p1/1
  k18/1 -> predefined/6(k2)
  k21/1 -> Product15/1
  Add46/1 -> Add47/1
  Add45/1 -> tua13/1
  psi12/1 -> To Workspace95/1, show_v psi gamma24/1, MATLAB Function22/5(psi), X_dot6/4(psi), U/4(psi)
  tua14/1 -> show_tua/2, predefined/17(tua2), Product14/2
  z0x6/1 -> MATLAB Function24/3(z0x)
  psi_r11/1 -> psi_r12/2
  z2y6/1 -> predefined/14(z2y), Add42/1, show_v psi gamma22/2, MATLAB Function21/5(z2y)
  predefined/3(nta_3) -> Add39/2, qnta/3(nta3)
  sys/8(s2) -> show_s/2, predefined/11(p2y)
  sys/9(s3) -> show_s/3, predefined/12(p2z)
  qnta/2(qnta2) -> Add46/1, show_qnta/2, U/8(qnta_2)
  zr11/1 -> zr12/2
  MATLAB Function22/1(dx) -> Add41/2, show_v psi gamma21/1, d2x 6/1
  gamma_r11/1 -> ref_UAV/6(gamma_r), X_dot6/3(gamma_r)
  z2z6/1 -> Add43/1, show_v psi gamma23/2, predefined/15(z2z), MATLAB Function23/5(z2z)
  X_dot6/3(dz) -> sys/5(dz), z12/1
  omiga_psi_r6/1 -> ref_UAV/3(omiga_psi_r), psi_r12/1
  gamma_r12/1 -> gamma_r11/2
  predefined/2(nta_2) -> Add46/2, qnta/2(nta2)
  U/2(u2_omiga_gamma) -> To Workspace93/1, show_u/2, gamma12/1
  z1y6/1 -> MATLAB Function21/4(z1y)
  U/3(u3_a) -> v12/1, To Workspace94/1, show_u/3
  ref_UAV/2(a_yr) -> U/2(a_yr), predefined/20(a_yr)
  x12/1 -> To Workspace91/1, uav_position/1, sys/2(x)
  gamma12/1 -> MATLAB Function22/4(gamma), show_v psi gamma24/2, To Workspace96/1, X_dot6/5(gamma), U/5(gamma)
  X_dot6/1(dx) -> sys/1(dx), x12/1
  MATLAB Function22/2(dy) -> d2y 6/1, Add42/2, show_v psi gamma22/1
  sys/2(p1y) -> MATLAB Function21/1(p1y), predefined/8(p1y), To Workspace103/1, show_p1/2
  " a^r4"/3(a_zr) -> control input 4/3(a_zr)
  f,df4/7(s1) -> yuding_zhishu4/10(p2x), p21/1
  Add12/1 -> To Workspace55/1, p19/3
  z7/1 -> z8/2
  t4/1 -> yuding_zhishu4/1(t)
  f,df4/5(p2y) -> MATLAB Function13/2(p2y), p23/2
  MATLAB Function16/2(dz1x) -> z1x4/1
  X_dot4/5(yr_dot) -> yr8/1, f,df4/9(dyr)
  z0y4/1 -> MATLAB Function13/3(z0y)
  psi7/1 -> psi8/2
  bta4/1 -> yuding_zhishu4/4(bta2), yuding_zhishu4/3(bta1)
  control input 4/2(u2_omiga_gamma) -> To Workspace58/1, show_u7/2, gamma8/1
  yuding_zhishu4/3(nta_3) -> control input 4/9(nta_3)
  MATLAB Function14/3(dz) -> Add12/2, show_v psi gamma15/1, d2z 4/1
  f,df4/1(p1x) -> MATLAB Function16/1(p1x), yuding_zhishu4/7(p1x), To Workspace66/1, p22/1
  control input 4/3(u3_a) -> v8/1, To Workspace59/1, show_u7/3
  f,df4/9(s3) -> yuding_zhishu4/12(p2z), p21/3
  d2y 4/1 -> p24/2, f,df4/14(wy), X_dot4/8(wy)
  Add11/1 -> To Workspace64/1, p19/2
  Add10/1 -> To Workspace63/1, p19/1
  " a^r4"/2(a_yr) -> control input 4/2(a_yr)
  zr7/1 -> zr8/2
  yr7/1 -> yr8/2
  MATLAB Function15/3(dz2z) -> z2z4/1
  MATLAB Function15/1(dz0z) -> z0z4/1
  ar4/1 -> " a^r4"/1(ar), vr8/1
  f,df4/2(p1y) -> MATLAB Function13/1(p1y), yuding_zhishu4/8(p1y), To Workspace67/1, p22/2
  psi_r8/1 -> X_dot4/2(psi_r), " a^r4"/4(psi_r)
  z8/1 -> To Workspace71/1, X4/3, f,df4/6(z)
  MATLAB Function14/2(dy) -> d2y 4/1, Add11/2, show_v psi gamma14/1
  y7/1 -> y8/2
  vr7/1 -> vr8/2
  z2z4/1 -> Add12/1, show_v psi gamma15/2, MATLAB Function15/5(z2z), yuding_zhishu4/15(z2z)
  vr8/1 -> X_dot4/1(vr), " a^r4"/2(vr)
  z2x4/1 -> Add10/1, show_v psi gamma13/2, MATLAB Function16/5(z2x), yuding_zhishu4/13(z2x)
  f,df4/6(p2z) -> MATLAB Function15/2(p2z), p23/3
  gamma_r8/1 -> gamma_r7/2
  X_dot4/6(zr_dot) -> f,df4/11(dzr), zr8/1
  MATLAB Function14/1(dx) -> Add10/2, show_v psi gamma13/1, d2x 4/1
  z2y4/1 -> MATLAB Function13/5(z2y), Add11/1, show_v psi gamma14/2, yuding_zhishu4/14(z2y)
  gamma_r7/1 -> " a^r4"/6(gamma_r), X_dot4/3(gamma_r)
  Clock4/1 -> MATLAB Function14/1(t)
  X_dot4/1(s1) -> f,df4/1(dx), x8/1
  k4/1 -> yuding_zhishu4/6(k2), yuding_zhishu4/5(k1)
  z1y4/1 -> MATLAB Function13/4(z1y)
  xr8/1 -> To Workspace68/1, show Xr4/1, f,df4/8(xr)
  z1x4/1 -> MATLAB Function16/4(z1x)
  MATLAB Function16/3(dz2x) -> z2x4/1
  gamma8/1 -> MATLAB Function14/4(gamma), show_v psi gamma16/2, To Workspace61/1, X_dot4/5(gamma), control input 4/5(gamma)
  xr7/1 -> xr8/2
  d2x 4/1 -> f,df4/13(wx), X_dot4/7(wx), p24/1
  z0x4/1 -> MATLAB Function16/3(z0x)
  zr8/1 -> To Workspace72/1, show Xr4/3, f,df4/12(zr)
  X_dot4/3(s3) -> f,df4/5(dz), z8/1
  d2z 4/1 -> f,df4/15(wz), X_dot4/9(wz), p20/2, p24/3
  Gain4/1 -> MATLAB Function14/2(delta)
  X_dot4/2(s2) -> y8/1, f,df4/3(dy)
  MATLAB Function13/1(dz0y) -> z0y4/1
  psi8/1 -> To Workspace60/1, show_v psi gamma16/1, MATLAB Function14/5(psi), X_dot4/4(psi), control input 4/4(psi)
  f,df4/8(s2) -> yuding_zhishu4/11(p2y), p21/2
  x7/1 -> x8/2
  control input 4/1(u1_omiga_psi) -> psi8/1, To Workspace57/1, show_u7/1
  z1z4/1 -> MATLAB Function15/4(z1z), p20/1
  yuding_zhishu4/2(nta_2) -> control input 4/8(nta_2)
  psi_r7/1 -> psi_r8/2
  omiga_psi_r4/1 -> " a^r4"/3(omiga_psi_r), psi_r8/1
  z0z4/1 -> MATLAB Function15/3(z0z)
  gamma7/1 -> gamma8/2
  MATLAB Function16/1(dz0x) -> z0x4/1
  f,df4/3(p1z) -> MATLAB Function15/1(p1z), yuding_zhishu4/9(p1z), To Workspace69/1, p22/3
  y8/1 -> To Workspace65/1, X4/2, f,df4/4(y)
  x8/1 -> To Workspace56/1, X4/1, f,df4/2(x)
  f,df4/4(p2x) -> MATLAB Function16/2(p2x), p23/1
  yuding_zhishu4/1(nta_1) -> control input 4/7(nta_1)
  MATLAB Function15/2(dz1z) -> z1z4/1
  v8/1 -> MATLAB Function14/3(v), To Workspace62/1, show_v psi gamma16/3, X_dot4/6(v), show_u8/1, control input 4/6(v)
  MATLAB Function13/3(dz2y) -> z2y4/1
  MATLAB Function13/2(dz1y) -> z1y4/1
  " a^r4"/1(a_xr) -> control input 4/1(a_xr)
  t_f4/1 -> yuding_zhishu4/2(t_f)
  yr8/1 -> To Workspace70/1, show Xr4/2, f,df4/10(yr)
  omiga__gamma_r4/1 -> " a^r4"/5(omiga_gamma_r), gamma_r7/1
  v7/1 -> v8/2
  X_dot4/4(xr_dot) -> f,df4/7(dxr), xr8/1
  Band-Limited White Noise4/1 -> Gain4/1
  MATLAB Function20/2(dz1y) -> z1y5/1
  u_2a6/1(u_2a) -> To Workspace76/1, show_u9/2, gamma10/1
  t_f5/1 -> yuding_zhishu5/2(t_f)
  X_dot5/5(yr_dot) -> yr10/1, f,df5/9(dyr)
  Clock5/1 -> MATLAB Function17/1(t)
  ar5/1 -> " a^r5"/1(ar), vr10/1
  f,df5/5(p2y) -> MATLAB Function20/2(p2y), p35/2
  z2x5/1 -> Add13/1, show_v psi gamma20/2, yuding_zhishu5/13(z2x), MATLAB Function19/5(z2x)
  f,df5/1(p1x) -> MATLAB Function19/1(p1x), yuding_zhishu5/7(p1x), To Workspace84/1, p28/1
  gamma10/1 -> MATLAB Function17/4(gamma), show_v psi gamma19/2, To Workspace79/1, X_dot5/5(gamma), control input 5/5(gamma)
  f,df5/6(p2z) -> MATLAB Function18/2(p2z), p35/3
  psi10/1 -> To Workspace78/1, show_v psi gamma19/1, MATLAB Function17/5(psi), X_dot5/4(psi), control input 5/4(psi)
  omiga__gamma_r5/1 -> " a^r5"/5(omiga_gamma_r), gamma_r9/1
  d2y 5/1 -> p36/2, f,df5/14(wy), X_dot5/8(wy)
  bta5/1 -> yuding_zhishu5/4(bta2), yuding_zhishu5/3(bta1)
  psi_r10/1 -> X_dot5/2(psi_r), " a^r5"/4(psi_r)
  xr10/1 -> To Workspace86/1, show Xr5/1, f,df5/8(xr)
  d2z 6/1 -> f,df5/15(wz), X_dot5/9(wz), p26/2, p36/3
  Add13/1 -> To Workspace81/1, p25/1
  " a^r5"/1(a_xr) -> control input 5/1(a_xr)
  xr9/1 -> xr10/2
  MATLAB Function19/3(dz2x) -> z2x5/1
  MATLAB Function17/1(dx) -> Add13/2, show_v psi gamma20/1, d2x 5/1
  f,df5/8(s2) -> yuding_zhishu5/11(p2y), p27/2
  psi9/1 -> psi10/2
  MATLAB Function19/2(dz1x) -> z1x5/1
  z0z5/1 -> MATLAB Function18/3(z0z)
  " a^r5"/2(a_yr) -> control input 5/2(a_yr)
  Band-Limited White Noise5/1 -> Gain5/1
  gamma_r9/1 -> " a^r5"/6(gamma_r), X_dot5/3(gamma_r)
  MATLAB Function17/3(dz) -> Add15/2, show_v psi gamma18/1, d2z 6/1
  yuding_zhishu5/2(nta_2) -> control input 5/8(nta_2)
  gamma_r10/1 -> gamma_r9/2
  v10/1 -> sat_v2/1
  control input 5/1(u1_omiga_psi) -> u_1a5/1(u)
  y10/1 -> To Workspace83/1, X5/2, f,df5/4(y)
  psi_r9/1 -> psi_r10/2
  z2y5/1 -> Add14/1, show_v psi gamma17/2, yuding_zhishu5/14(z2y), MATLAB Function20/5(z2y)
  Gain5/1 -> MATLAB Function17/2(delta)
  control input 5/3(u3_a) -> u_3a5/1(u)
  X_dot5/3(s3) -> f,df5/5(dz), z10/1
  MATLAB Function18/3(dz2z) -> z2z5/1
  MATLAB Function18/2(dz1z) -> z1z5/1
  MATLAB Function18/1(dz0z) -> z0z5/1
  u_1a5/1(u_1a) -> psi10/1, To Workspace75/1, show_u9/1
  z1z5/1 -> p26/1, MATLAB Function18/4(z1z)
  z0y5/1 -> MATLAB Function20/3(z0y)
  " a^r5"/3(a_zr) -> control input 5/3(a_zr)
  z2z5/1 -> Add15/1, show_v psi gamma18/2, yuding_zhishu5/15(z2z), MATLAB Function18/5(z2z)
  MATLAB Function20/1(dz0y) -> z0y5/1
  x10/1 -> To Workspace74/1, X5/1, f,df5/2(x)
  z0x5/1 -> MATLAB Function19/3(z0x)
  Add15/1 -> To Workspace73/1, p25/3
  X_dot5/2(s2) -> y10/1, f,df5/3(dy)
  X_dot5/4(xr_dot) -> f,df5/7(dxr), xr10/1
  zr10/1 -> To Workspace90/1, show Xr5/3, f,df5/12(zr)
  x9/1 -> x10/2
  X_dot5/6(zr_dot) -> f,df5/11(dzr), zr10/1
  MATLAB Function17/2(dy) -> d2y 5/1, Add14/2, show_v psi gamma17/1
  yuding_zhishu5/3(nta_3) -> control input 5/9(nta_3)
  gamma9/1 -> gamma10/2
  f,df5/4(p2x) -> MATLAB Function19/2(p2x), p35/1
  t5/1 -> yuding_zhishu5/1(t)
  X_dot5/1(s1) -> f,df5/1(dx), x10/1
  Add14/1 -> To Workspace82/1, p25/2
  sat_v2/1 -> MATLAB Function17/3(v), To Workspace80/1, show_v psi gamma19/3, X_dot5/6(v), show_u10/1, control input 5/6(v)
  f,df5/9(s3) -> yuding_zhishu5/12(p2z), p27/3
  omiga_psi_r5/1 -> " a^r5"/3(omiga_psi_r), psi_r10/1
  yr10/1 -> To Workspace88/1, show Xr5/2, f,df5/10(yr)
  MATLAB Function20/3(dz2y) -> z2y5/1
  z1x5/1 -> MATLAB Function19/4(z1x)
  f,df5/7(s1) -> yuding_zhishu5/10(p2x), p27/1
  f,df5/3(p1z) -> MATLAB Function18/1(p1z), yuding_zhishu5/9(p1z), To Workspace87/1, p28/3
  control input 5/2(u2_omiga_gamma) -> u_2a6/1(u)
  u_3a5/1(u_3a) -> v10/1, To Workspace77/1, show_u9/3
  f,df5/2(p1y) -> MATLAB Function20/1(p1y), yuding_zhishu5/8(p1y), To Workspace85/1, p28/2
  vr9/1 -> vr10/2
  yr9/1 -> yr10/2
  y9/1 -> y10/2
  v9/1 -> v10/2
  k5/1 -> yuding_zhishu5/5(k1)
  z10/1 -> To Workspace89/1, X5/3, f,df5/6(z)
  MATLAB Function19/1(dz0x) -> z0x5/1
  z9/1 -> z10/2
  vr10/1 -> X_dot5/1(vr), " a^r5"/2(vr)
  yuding_zhishu5/1(nta_1) -> control input 5/7(nta_1)
  zr9/1 -> zr10/2
  d2x 5/1 -> f,df5/13(wx), X_dot5/7(wx), p36/1
  z1y5/1 -> MATLAB Function20/4(z1y)
  k7/1 -> predefined/5(k1)
  k8/1 -> yuding_zhishu3/6(k2)
  k9/1 -> yuding_zhishu5/6(k2)

== matlab function paper_Exponential_Predefined_102/ a^r1 ==
  data: ar input; vr input; a_xr output; a_yr output; omiga_psi_r input; psi_r input; omiga_gamma_r input; a_zr output; gamma_r input
function [a_xr,a_yr,a_zr] = fcn(ar,vr,omiga_psi_r,psi_r,omiga_gamma_r,gamma_r)
a_xr = -vr*sin(psi_r)*cos(gamma_r)*omiga_psi_r-vr*cos(psi_r)*sin(gamma_r)*omiga_gamma_r+cos(psi_r)*cos(gamma_r)*ar;
a_yr = vr*cos(psi_r)*cos(gamma_r)*omiga_psi_r-vr*sin(psi_r)*sin(gamma_r)*omiga_gamma_r+ sin(psi_r)*cos(gamma_r)*ar;
a_zr = vr*cos(gamma_r)*omiga_gamma_r + sin(gamma_r)*ar;
end

== matlab function paper_Exponential_Predefined_102/MATLAB Function1 ==
  data: p1y input; p2y input; z0y input; dz0y output; dz1y output; dz2y output; z1y input; z2y input
function [dz0y,dz1y,dz2y] = FTDO(p1y,p2y,z0y,z1y,z2y)
r=[24 216 864];
r0=r(1);
r1=r(2);
r2=r(3);
v0=-r0*(abs(z0y-p1y))^(0.8)*sign(z0y-p1y)-r0*(abs(z0y-p1y))^(1.2)*sign(z0y-p1y)+z1y;
dz0y=v0+p2y;
v1=-r1*(abs(z0y-p1y))^(0.6)*sign(z0y-p1y)-r1*(abs(z0y-p1y))^(1.4)*sign(z0y-p1y)+z2y;
dz1y=v1;
dz2y =-r2*(abs(z0y-p1y))^(0.4)*sign(z0y-p1y)-r2*(abs(z0y-p1y))^(1.6)*sign(z0y-p1y);
end

== matlab function paper_Exponential_Predefined_102/MATLAB Function2 ==
  data: t input; dx output; dy output; dz output; delta input; v input; gamma input; psi input
function [dx,dy,dz] = disturbance(t,delta,v,gamma,psi)
fx=-0.0005*abs(v-36)*exp((0.4*v)^0.5)+0.2*sin(psi);
fy=-0.0004*abs(v-30)*exp((0.3*v)^0.5)+0.2*cos(psi);
fz=-0.004*v^(0.5)*sin(3*gamma);
% fx=0;
% fy=0;
% fz=0;
if 0<t && t<10
    wx = 1*sin(t)+delta;
else
    wx=0;
end
if 5<t && t<15
    wy = 2*sin(2*t)-cos(3*t)+delta;
else
    wy=0;
end
if 0<t && t<20
    wz = 0.5*sin(t)+delta;
else
    wz = 0;
end

dx=fx+wx;
dy=fy+wy;
dz=fz+wz;

end

== matlab function paper_Exponential_Predefined_102/MATLAB Function3 ==
  data: p1z input; p2z input; z0z input; dz0z output; dz1z output; dz2z output; z1z input; z2z input
function [dz0z,dz1z,dz2z] = FTDO(p1z,p2z,z0z,z1z,z2z)
r=[24 216 864];
r0=r(1);
r1=r(2);
r2=r(3);
v0=-r0*(abs(z0z-p1z))^(0.8)*sign(z0z-p1z)-r0*(abs(z0z-p1z))^(1.2)*sign(z0z-p1z)+z1z;
dz0z=v0+p2z;
v1=-r1*(abs(z0z-p1z))^(0.6)*sign(z0z-p1z)-r1*(abs(z0z-p1z))^(1.4)*sign(z0z-p1z)+z2z;
dz1z=v1;
dz2z =-r2*(abs(z0z-p1z))^(0.4)*sign(z0z-p1z)-r2*(abs(z0z-p1z))^(1.6)*sign(z0z-p1z);
end

== matlab function paper_Exponential_Predefined_102/MATLAB Function4 ==
  data: p1x input; p2x input; z0x input; dz0x output; dz1x output; dz2x output; z1x input; z2x input
function [dz0x,dz1x,dz2x] = FTDO(p1x,p2x,z0x,z1x,z2x)
r=[24 216 864];%parameters of FTDO
r0=r(1);
r1=r(2);
r2=r(3);
v0=-r0*(abs(z0x-p1x))^(0.8)*sign(z0x-p1x)-r0*(abs(z0x-p1x))^(1.2)*sign(z0x-p1x)+z1x;
dz0x=v0+p2x;
v1=-r1*(abs(z0x-p1x))^(0.6)*sign(z0x-p1x)-r1*(abs(z0x-p1x))^(1.4)*sign(z0x-p1x)+z2x;
dz1x=v1;
dz2x =-r2*(abs(z0x-p1x))^(0.4)*sign(z0x-p1x)-r2*(abs(z0x-p1x))^(1.6)*sign(z0x-p1x);
end

== matlab function paper_Exponential_Predefined_102/X_dot1 ==
  data: vr input; psi_r input; gamma_r input; psi input; gamma input; v input; s1 output; s2 output; s3 output; xr_dot output; yr_dot output; zr_dot output; wx input; wy input; wz input
function [s1,s2,s3,xr_dot,yr_dot,zr_dot] = fcn(vr,psi_r,gamma_r,psi,gamma,v,wx,wy,wz)
wx=0;
wy=0;
wz=0;
s1 = v*cos(psi)*cos(gamma)+wx;
s2 = v*sin(psi)*cos(gamma)+wy;
s3 = v*sin(gamma)+wz;
xr_dot = vr*cos(psi_r)*cos(gamma_r);
yr_dot = vr*sin(psi_r)*cos(gamma_r);
zr_dot = vr*sin(gamma_r);
end

== matlab function paper_Exponential_Predefined_102/control input 1 ==
  data: a_xr input; a_yr input; a_zr input; psi input; gamma input; u1_omiga_psi output; u2_omiga_gamma output; u3_a output; v input; nta_1 input; nta_2 input; nta_3 input
function [u1_omiga_psi,u2_omiga_gamma,u3_a] = fcn(a_xr,a_yr,a_zr,psi,gamma,v,nta_1,nta_2,nta_3)
A = [-a_xr;-a_yr;-a_zr];
B = [-v*sin(psi)*cos(gamma) -v*cos(psi)*sin(gamma) cos(psi)*cos(gamma); 
    v*cos(psi)*cos(gamma) -v*sin(psi)*sin(gamma) sin(psi)*cos(gamma);
    0                        v*cos(gamma)               sin(gamma)];
nta = [nta_1 ; nta_2;nta_3];
U = -inv(B)*(A - nta);
U11=U(1,1); 
U21=U(2,1);
U31=U(3,1);
% 

u1_omiga_psi = U11 ;
u2_omiga_gamma = U21;
u3_a =U31 ;






end

== matlab function paper_Exponential_Predefined_102/f,df1 ==
  data: dx input; x input; dy input; y input; dz input; z input; dxr input; xr input; dyr input; yr input; dzr input; zr input; p1x output; p1y output; p1z output; p2x output; p2y output; p2z output; wx input; wy input; wz input; s1 output; s2 output; s3 output
 function [p1x,p1y,p1z,p2x,p2y,p2z,s1,s2,s3] = fcn(dx,x,dy,y,dz,z,dxr,xr,dyr,yr,dzr,zr,wx,wy,wz)
wx=0;
wy=0;
wz=0;
p1x = x - xr;
p1y = y - yr;
p1z = z - zr;
s1 = dx - dxr ;
s2 = dy - dyr ;
s3 = dz - dzr ;%w为了确保输入的p2是没有包含扰动的，这样估计值才会准
p2x = dx - dxr-wx ;
p2y = dy - dyr-wy ;
p2z = dz - dzr-wz ;
end

== matlab function paper_Exponential_Predefined_102/ a^r2 ==
  data: ar input; vr input; a_xr output; a_yr output; omiga_psi_r input; psi_r input; omiga_gamma_r input; a_zr output; gamma_r input
function [a_xr,a_yr,a_zr] = fcn(ar,vr,omiga_psi_r,psi_r,omiga_gamma_r,gamma_r)
a_xr = -vr*sin(psi_r)*cos(gamma_r)*omiga_psi_r-vr*cos(psi_r)*sin(gamma_r)*omiga_gamma_r+cos(psi_r)*cos(gamma_r)*ar;
a_yr = vr*cos(psi_r)*cos(gamma_r)*omiga_psi_r-vr*sin(psi_r)*sin(gamma_r)*omiga_gamma_r+ sin(psi_r)*cos(gamma_r)*ar;
a_zr = vr*cos(gamma_r)*omiga_gamma_r + sin(gamma_r)*ar;
end

== matlab function paper_Exponential_Predefined_102/u_1a2 ==
  data: u input; u_1a output
function u_1a  = fcn(u)

u_max=1;

u_1a=u_max*erf((pi^(0.5)*u)/(2*u_max));


 end

== matlab function paper_Exponential_Predefined_102/u_2a1 ==
  data: u input; u_2a output
function u_2a  = fcn(u)

u_max=1;

u_2a=u_max*erf((pi^(0.5)*u)/(2*u_max));


 end

== matlab function paper_Exponential_Predefined_102/u_3a1 ==
  data: u input; u_3a output
function u_3a  = fcn(u)

u_max=10;
v_max=15;
% u_3a=u;
u_3a=u_max*erf((pi^(0.5)*u)/(2*u_max));
% q_v=erf((pi^(0.5)*(v-25))/(2*v_max));
% % u_3a=q_u*(1-abs(q_v));
% if v>=40 & u>0
%     u_3a=0;
% elseif v<=10 & u<0
%     u_3a=0;
% else
%     u_3a=u_max*erf((pi^(0.5)*u)/(2*u_max));
    
 end
